simulink model "Ans_2H"  (R2021a)
settings: Solver=VariableStepAuto  StartTime=0.0  StopTime=1  RelTol=1e-3
values from neighbouring files (symbols this model uses):
  A_act = [0  1; -22500  -210]    [Ans_2_F.mat]
  A_s = [0  0; 0  0]    [Ans_2_F.mat]
  B_act = [0 22500]    [Ans_2_F.mat]
  B_s = [0  0; 0  0]    [Ans_2_F.mat]
  C_act = [1 0]    [Ans_2_F.mat]
  C_s = [0  0; 0  0]    [Ans_2_F.mat]
  D_act = 0    [Ans_2_F.mat]
  D_s = [1  0; 0  1]    [Ans_2_F.mat]
  Unitgain = 1    [Ans_2_F.mat]
undefined symbols (not defined in the file or in its folder): K_q, K_sc, Kprime_cf_red, Kprime_dr_red, T_rm
libraries: RCTblocks x1, simulink_extras x1
settings Model: LastModifiedBy=s347520

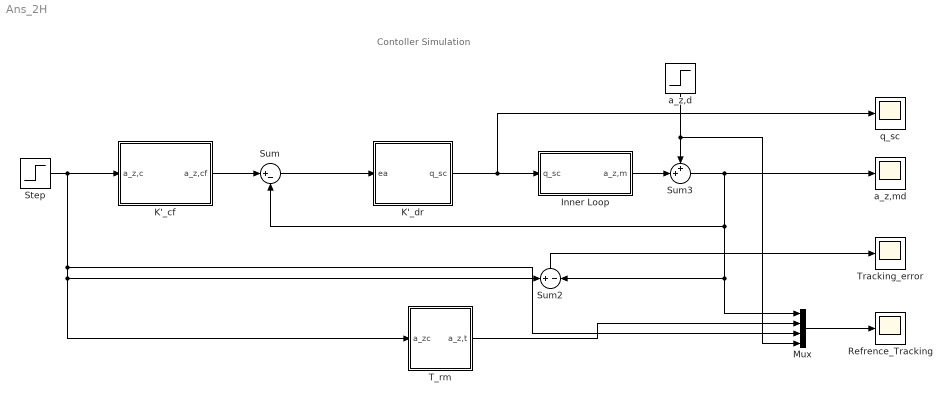
== system Ans_2H ==
  note: Contoller Simulation
  Inner Loop : Subsystem
  K'_cf : Subsystem
  K'_dr : Subsystem
  Mux : Mux
  Refrence_Tracking : Scope
  Step : Step  Time=0  SampleTime=0
  Sum : Sum  Inputs=|+-
  Sum2 : Sum  Inputs=+|-
  Sum3 : Sum  Inputs=++|
  T_rm : Subsystem
  Tracking_error : Scope
  a_z,d : Step  Time=0.2  After=0.1  SampleTime=0
  a_z,md : Scope
  q_sc : Scope
  wires:
  K'_cf/1(a_z,cf) -> Sum/1
  Step/1 -> Mux/3, T_rm/1(a_zc), Sum2/1, K'_cf/1(a_z,c)
  Mux/1 -> Refrence_Tracking/1
  Sum/1 -> K'_dr/1(ea)
  T_rm/1(a_z,t) -> Mux/2
  Sum2/1 -> Tracking_error/1
  Inner Loop/1(a_z,m) -> Sum3/2
  Sum3/1 -> Sum/2, Sum2/2, Mux/1, a_z,md/1
  a_z,d/1 -> Mux/4, Sum3/1
  K'_dr/1(q_sc) -> q_sc/1, Inner Loop/1(q_sc)

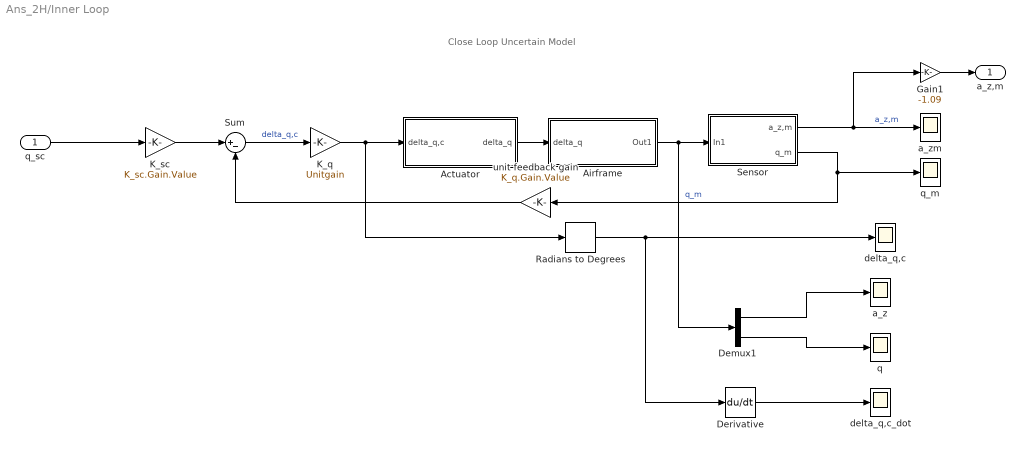
== system Ans_2H/Inner Loop ==
  note: Close Loop Uncertain Model
  q_sc : Inport
  Actuator : Subsystem
  Airframe : Subsystem
  Demux1 : Demux  Outputs=2
  Derivative : Derivative
  Gain1 : Gain  Gain=-1.09
  K_q : Gain  Gain=Unitgain
  K_sc : Gain  Gain=K_sc.Gain.Value
  Radians to Degrees : simulink_extras/Transformations/Radians to Degrees
  Sensor : Subsystem
  Sum : Sum  Inputs=|+-
  a_z : Scope
  a_zm : Scope
  delta_q,c : Scope
  delta_q,c_dot : Scope
  q : Scope
  q_m : Scope
  unit feedback gain : Gain  Gain=K_q.Gain.Value
  a_z,m : Outport
  wires:
  Sensor/1(a_z,m) -> Gain1/1, a_zm/1  "a_z,m"
  Airframe/1(Out1) -> Demux1/1, Sensor/1(In1)
  Radians to Degrees/1 -> Derivative/1, delta_q,c/1
  Demux1/2 -> q/1
  Sum/1 -> K_q/1  "delta_q,c"
  q_sc/1 -> K_sc/1
  K_sc/1 -> Sum/1
  Sensor/2(q_m) -> unit feedback gain/1, q_m/1  "q_m"
  Actuator/1(delta_q) -> Airframe/1(delta_q)
  Demux1/1 -> a_z/1
  Derivative/1 -> delta_q,c_dot/1
  unit feedback gain/1 -> Sum/2
  Gain1/1 -> a_z,m/1
  K_q/1 -> Actuator/1(delta_q,c), Radians to Degrees/1

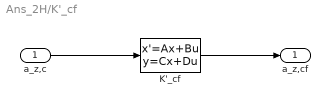
== system Ans_2H/K'_cf ==
  a_z,c : Inport
  K'_cf : StateSpace  A=Kprime_cf_red.A  B=Kprime_cf_red.B  C=Kprime_cf_red.C  D=Kprime_cf_red.D  InitialCondition=0
  a_z,cf : Outport
  wires:
  K'_cf/1 -> a_z,cf/1
  a_z,c/1 -> K'_cf/1

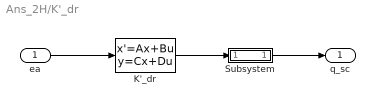
== system Ans_2H/K'_dr ==
  ea : Inport
  K'_dr : StateSpace  A=Kprime_dr_red.A  B=Kprime_dr_red.B  C=Kprime_dr_red.C  D=Kprime_dr_red.D  InitialCondition=0
  Subsystem : Subsystem
  q_sc : Outport
  wires:
  ea/1 -> K'_dr/1
  K'_dr/1 -> Subsystem/1(In1)
  Subsystem/1(Out1) -> q_sc/1

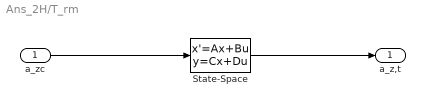
== system Ans_2H/T_rm ==
  a_zc : Inport
  State-Space : StateSpace  A=T_rm.A  B=T_rm.B  C=T_rm.C  D=T_rm.D  InitialCondition=0  ParameterTunability=Unconstrained
  a_z,t : Outport
  wires:
  State-Space/1 -> a_z,t/1
  a_zc/1 -> State-Space/1

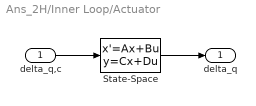
== system Ans_2H/Inner Loop/Actuator ==
  delta_q,c : Inport
  State-Space : StateSpace  A=A_act  B=B_act  C=C_act  D=D_act  InitialCondition=0
  delta_q : Outport
  wires:
  State-Space/1 -> delta_q/1
  delta_q,c/1 -> State-Space/1

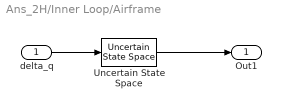
== system Ans_2H/Inner Loop/Airframe ==
  delta_q : Inport
  Uncertain State Space : RCTblocks/Uncertain State Space  Tag=USS  USystem=G_un  UValue=G_un.Uncertainty  X0=[]  uX0=[]
      settings: SourceProductBaseCode=RC
  Out1 : Outport
  wires:
  delta_q/1 -> Uncertain State Space/1
  Uncertain State Space/1 -> Out1/1

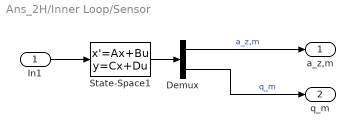
== system Ans_2H/Inner Loop/Sensor ==
  In1 : Inport
  Demux : Demux  Outputs=2
  State-Space1 : StateSpace  A=A_s  B=B_s  C=C_s  D=D_s  InitialCondition=0
  a_z,m : Outport
  q_m : Outport  Port=2
  wires:
  In1/1 -> State-Space1/1
  State-Space1/1 -> Demux/1
  Demux/1 -> a_z,m/1  "a_z,m"
  Demux/2 -> q_m/1  "q_m"

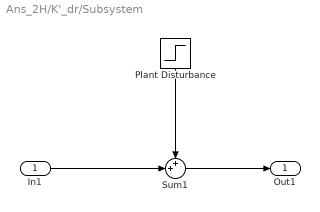
== system Ans_2H/K'_dr/Subsystem ==
  In1 : Inport
  Plant Disturbance : Step  Time=0  After=0.1  SampleTime=0
  Sum1 : Sum  Inputs=++|
  Out1 : Outport
  wires:
  Plant Disturbance/1 -> Sum1/1
  In1/1 -> Sum1/2
  Sum1/1 -> Out1/1
